simulink model "Powertrain_Mechanics_and_Dynamics"  (R2017b)
settings: Solver=VariableStepAuto  StartTime=0.0  StopTime=5  RelTol=1e-3
values from neighbouring files (symbols this model uses):
  P_2_0 = 0    [Gearbox_SLX_m.m]
  x_5_0 = 0    [Gearbox_SLX_m.m]
undefined symbols (not defined in the file or in its folder): A, b_dt, b_r, b_rg, C_d, c_roll, g, J_dt, J_r, K_dt, K_rg, M, P_3_0, P_4_0, r_g, r_r, r_w, rho, slope_out, w_6_0, x_in
settings Model: Creator=Luca  LastModifiedBy=Luca

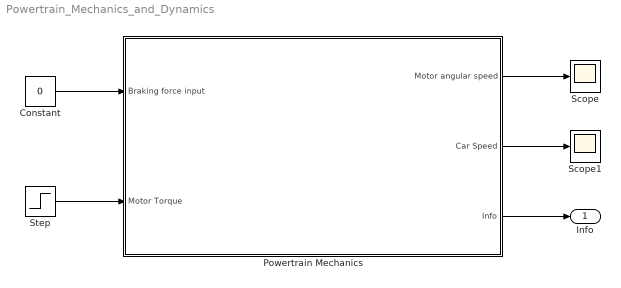
== system Powertrain_Mechanics_and_Dynamics ==
  Constant : Constant  Value=0
  Powertrain Mechanics : Subsystem
  Scope : Scope
  Scope1 : Scope
  Step : Step  After=200  SampleTime=0
  Info : Outport
  wires:
  Constant/1 -> Powertrain Mechanics/1(Braking force input)
  Step/1 -> Powertrain Mechanics/2(Motor Torque)
  Powertrain Mechanics/1(Motor angular speed) -> Scope/1
  Powertrain Mechanics/2(Car Speed) -> Scope1/1
  Powertrain Mechanics/3(Info) -> Info/1

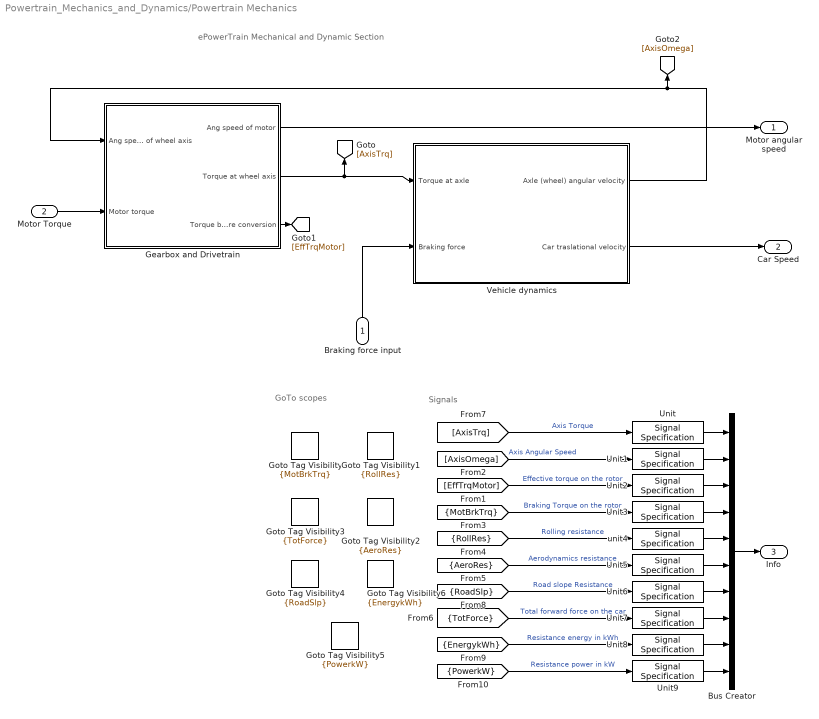
== system Powertrain_Mechanics_and_Dynamics/Powertrain Mechanics ==
  note: GoTo scopes
  note: Signals
  note: ePowerTrain Mechanical and Dynamic Section
  Braking force input : Inport
  Motor Torque : Inport  Port=2
  Bus Creator : BusCreator  Inputs=10
  Gearbox and Drivetrain : Subsystem
  Goto Tag Visibility : GotoTagVisibility  GotoTag=MotBrkTrq
  Goto Tag Visibility1 : GotoTagVisibility  GotoTag=RollRes
  Goto Tag Visibility2 : GotoTagVisibility  GotoTag=AeroRes
  Goto Tag Visibility3 : GotoTagVisibility  GotoTag=TotForce
  Goto Tag Visibility4 : GotoTagVisibility  GotoTag=RoadSlp
  Goto Tag Visibility5 : GotoTagVisibility  GotoTag=PowerkW
  Goto Tag Visibility6 : GotoTagVisibility  GotoTag=EnergykWh
  Unit : SignalSpecification  Unit=N*m
  Unit1 : SignalSpecification  Unit=rad/s
  Unit2 : SignalSpecification  Unit=N*m
  Unit3 : SignalSpecification  Unit=N*m
  Unit5 : SignalSpecification  Unit=N
  Unit6 : SignalSpecification  Unit=N
  Unit7 : SignalSpecification  Unit=N
  Unit8 : SignalSpecification  Unit=k*W*h
  Unit9 : SignalSpecification  Unit=k*W
  Vehicle dynamics : Subsystem
  unit4 : SignalSpecification  Unit=N
  Motor angular speed : Outport
  Car Speed : Outport  Port=2
  Info : Outport  Port=3
  wires:
  Vehicle dynamics/1(Axle (wheel) angular velocity) -> [AxisOmega], Gearbox and Drivetrain/1(Ang speed of wheel axis)
  Braking force input/1 -> Vehicle dynamics/2(Braking force)
  Gearbox and Drivetrain/2(Torque at wheel axis) -> Vehicle dynamics/1(Torque at axle), [AxisTrq]
  Gearbox and Drivetrain/3(Torque before conversion) -> [EffTrqMotor]
  [AxisOmega] -> Unit1/1  "Axis Angular Speed"
  [AxisTrq] -> Unit/1  "Axis Torque"
  Bus Creator/1 -> Info/1
  [RollRes] -> unit4/1  "Rolling resistance"
  Motor Torque/1 -> Gearbox and Drivetrain/2(Motor torque)
  Gearbox and Drivetrain/1(Ang speed of motor) -> Motor angular speed/1
  [AeroRes] -> Unit5/1  "Aerodynamics resistance"
  [MotBrkTrq] -> Unit3/1  "Braking Torque on the rotor"
  [TotForce] -> Unit7/1  "Total forward force on the car"
  [EffTrqMotor] -> Unit2/1  "Effective torque on the rotor"
  [RoadSlp] -> Unit6/1  "Road slope Resistance"
  Vehicle dynamics/2(Car traslational velocity) -> Car Speed/1
  [PowerkW] -> Unit9/1  "Resistance power in kW"
  [EnergykWh] -> Unit8/1  "Resistance energy in kWh"
  Unit/1 -> Bus Creator/1
  Unit1/1 -> Bus Creator/2
  Unit2/1 -> Bus Creator/3
  Unit3/1 -> Bus Creator/4
  unit4/1 -> Bus Creator/5
  Unit5/1 -> Bus Creator/6
  Unit6/1 -> Bus Creator/7
  Unit7/1 -> Bus Creator/8
  Unit8/1 -> Bus Creator/9
  Unit9/1 -> Bus Creator/10

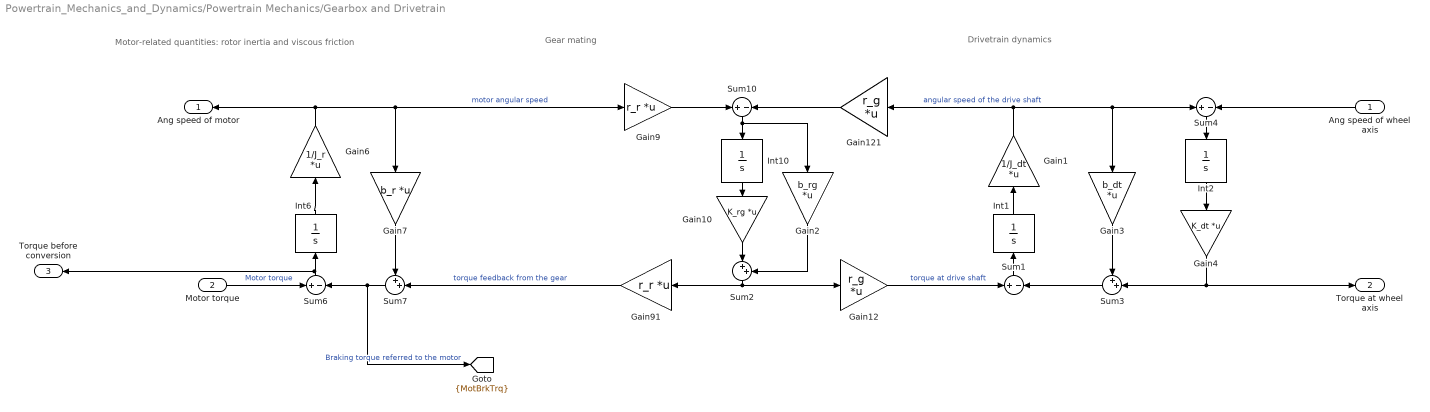
== system Powertrain_Mechanics_and_Dynamics/Powertrain Mechanics/Gearbox and Drivetrain ==
  note: Drivetrain dynamics
  note: Gear mating
  note: Motor-related quantities: rotor inertia and viscous friction
  Ang speed of wheel axis : Inport
  Motor torque : Inport  Port=2
  Gain1 : Gain  Gain=1/J_dt  Multiplication=Matrix(K*u)  SaturateOnIntegerOverflow=on  OutDataTypeStr=Inherit: Same as input  ParamDataTypeStr=Inherit: Same as input
  Gain10 : Gain  Gain=K_rg  Multiplication=Matrix(K*u)  SaturateOnIntegerOverflow=on  OutDataTypeStr=Inherit: Same as input  ParamDataTypeStr=Inherit: Same as input
  Gain12 : Gain  Gain=r_g  Multiplication=Matrix(K*u)  SaturateOnIntegerOverflow=on  OutDataTypeStr=Inherit: Same as input  ParamDataTypeStr=Inherit: Same as input
  Gain121 : Gain  Gain=r_g  Multiplication=Matrix(K*u)  SaturateOnIntegerOverflow=on  OutDataTypeStr=Inherit: Same as input  ParamDataTypeStr=Inherit: Same as input
  Gain2 : Gain  Gain=b_rg  Multiplication=Matrix(K*u)  SaturateOnIntegerOverflow=on  OutDataTypeStr=Inherit: Same as input  ParamDataTypeStr=Inherit: Same as input
  Gain3 : Gain  Gain=b_dt  Multiplication=Matrix(K*u)  SaturateOnIntegerOverflow=on  OutDataTypeStr=Inherit: Same as input  ParamDataTypeStr=Inherit: Same as input
  Gain4 : Gain  Gain=K_dt  Multiplication=Matrix(K*u)  SaturateOnIntegerOverflow=on  OutDataTypeStr=Inherit: Same as input  ParamDataTypeStr=Inherit: Same as input
  Gain6 : Gain  Gain=1/J_r  Multiplication=Matrix(K*u)  SaturateOnIntegerOverflow=on  OutDataTypeStr=Inherit: Same as input  ParamDataTypeStr=Inherit: Same as input
  Gain7 : Gain  Gain=b_r  Multiplication=Matrix(K*u)  SaturateOnIntegerOverflow=on  OutDataTypeStr=Inherit: Same as input  ParamDataTypeStr=Inherit: Same as input
  Gain9 : Gain  Gain=r_r  Multiplication=Matrix(K*u)  SaturateOnIntegerOverflow=on  OutDataTypeStr=Inherit: Same as input  ParamDataTypeStr=Inherit: Same as input
  Gain91 : Gain  Gain=r_r  Multiplication=Matrix(K*u)  SaturateOnIntegerOverflow=on  OutDataTypeStr=Inherit: Same as input  ParamDataTypeStr=Inherit: Same as input
  Int1 : Integrator  InitialCondition=P_3_0
  Int10 : Integrator  InitialCondition=x_5_0
  Int2 : Integrator  InitialCondition=w_6_0
  Int6 : Integrator  InitialCondition=P_2_0
  Sum{1,4,6,10} (4 alike) : Sum  Inputs=+|-  SaturateOnIntegerOverflow=on  InputSameDT=on  OutDataTypeStr=Inherit: Same as first input
  Sum2 : Sum  Inputs=|++  SaturateOnIntegerOverflow=on  InputSameDT=on  OutDataTypeStr=Inherit: Same as first input
  Sum3 : Sum  Inputs=++|  SaturateOnIntegerOverflow=on  InputSameDT=on  OutDataTypeStr=Inherit: Same as first input
  Sum7 : Sum  Inputs=++|  SaturateOnIntegerOverflow=on  InputSameDT=on  OutDataTypeStr=Inherit: Same as first input
  Ang speed of motor : Outport  VectorParamsAs1DForOutWhenUnconnected=on
  Torque at wheel axis : Outport  Port=2  VectorParamsAs1DForOutWhenUnconnected=on
  Torque before conversion : Outport  Port=3  VectorParamsAs1DForOutWhenUnconnected=on
  tag scope: MotBrkTrq=scoped
  wires:
  Gain91/1 -> Sum7/2  "torque feedback from the gear"
  Sum10/1 -> Gain2/1, Int10/1
  Gain6/1 -> Ang speed of motor/1, Gain9/1, Gain7/1  "motor angular speed"
  Sum7/1 -> [MotBrkTrq], Sum6/2  "Braking torque referred to the motor"
  Int6/1 -> Gain6/1
  Sum6/1 -> Torque before conversion/1, Int6/1
  Gain9/1 -> Sum10/1
  Gain7/1 -> Sum7/1
  Gain121/1 -> Sum10/2
  Sum2/1 -> Gain91/1, Gain12/1
  Gain10/1 -> Sum2/1
  Gain2/1 -> Sum2/2
  Motor torque/1 -> Sum6/1  "Motor torque"
  Int10/1 -> Gain10/1
  Gain12/1 -> Sum1/1  "torque at drive shaft"
  Sum3/1 -> Sum1/2
  Gain4/1 -> Sum3/2, Torque at wheel axis/1
  Int1/1 -> Gain1/1
  Sum1/1 -> Int1/1
  Gain1/1 -> Sum4/1, Gain3/1, Gain121/1  "angular speed of the drive shaft"
  Ang speed of wheel axis/1 -> Sum4/2
  Gain3/1 -> Sum3/1
  Int2/1 -> Gain4/1
  Sum4/1 -> Int2/1

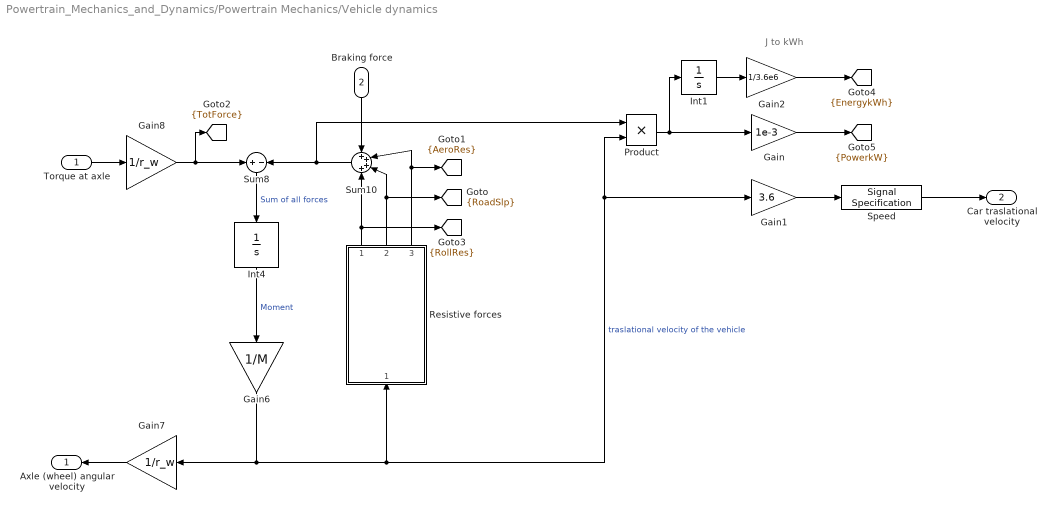
== system Powertrain_Mechanics_and_Dynamics/Powertrain Mechanics/Vehicle dynamics ==
  note: J to kWh
  Torque at axle : Inport
  Braking force : Inport  Port=2
  " Resistive forces" : Subsystem
  Gain : Gain  Gain=1e-3
  Gain1 : Gain  Gain=3.6
  Gain2 : Gain  Gain=1/3.6e6
  Gain6 : Gain  Gain=1/M  SaturateOnIntegerOverflow=on  OutDataTypeStr=Inherit: Same as input  ParamDataTypeStr=Inherit: Same as input
  Gain7 : Gain  Gain=1/r_w  SaturateOnIntegerOverflow=on  OutDataTypeStr=Inherit: Same as input  ParamDataTypeStr=Inherit: Same as input
  Gain8 : Gain  Gain=1/r_w  SaturateOnIntegerOverflow=on  OutDataTypeStr=Inherit: Same as input  ParamDataTypeStr=Inherit: Same as input
  Int1 : Integrator  InitialCondition=P_4_0
  Int4 : Integrator  InitialCondition=P_4_0
  Product : Product
  Speed : SignalSpecification  Unit=km/h
  Sum10 : Sum  Inputs=++++  SaturateOnIntegerOverflow=on  InputSameDT=on  OutDataTypeStr=Inherit: Same as first input
  Sum8 : Sum  Inputs=+|-  SaturateOnIntegerOverflow=on  InputSameDT=on  OutDataTypeStr=Inherit: Same as first input
  Axle (wheel) angular velocity : Outport
  Car traslational velocity : Outport  Port=2
  tag scope: AeroRes=scoped, EnergykWh=scoped, PowerkW=scoped, RoadSlp=scoped, RollRes=scoped, TotForce=scoped
  wires:
  Gain7/1 -> Axle (wheel) angular velocity/1
  Gain8/1 -> [TotForce], Sum8/1
  Sum8/1 -> Int4/1  "Sum of all forces"
  Gain6/1 -> Product/2, Gain1/1, " Resistive forces"/1(Traslational velocity), Gain7/1  "traslational velocity of the vehicle"
  Int4/1 -> Gain6/1  "Moment"
  Sum10/1 -> Product/1, Sum8/2
  Torque at axle/1 -> Gain8/1
  " Resistive forces"/2("  Road slope") -> Sum10/3, [RoadSlp]
  Braking force/1 -> Sum10/1
  " Resistive forces"/1(Rolling res) -> [RollRes], Sum10/4
  " Resistive forces"/3(" Drag Force") -> Sum10/2, [AeroRes]
  Product/1 -> Int1/1, Gain/1
  Int1/1 -> Gain2/1
  Gain1/1 -> Speed/1
  Speed/1 -> Car traslational velocity/1
  Gain2/1 -> [EnergykWh]
  Gain/1 -> [PowerkW]

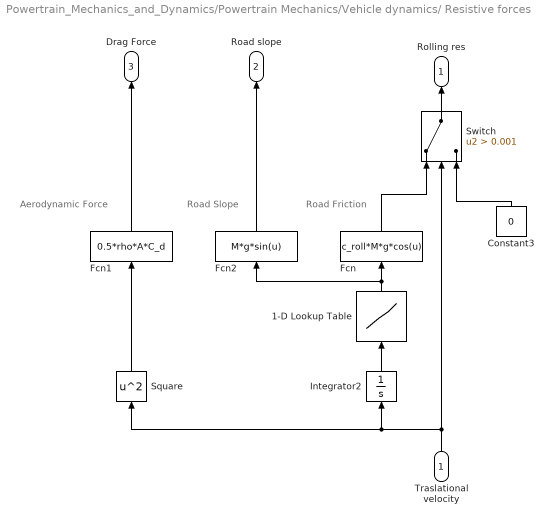
== system Powertrain_Mechanics_and_Dynamics/Powertrain Mechanics/Vehicle dynamics/ Resistive forces ==
  note: Aerodynamic Force
  note: Road Friction
  note: Road Slope
  Traslational velocity : Inport
  1-D Lookup Table : Lookup_n-D  NumberOfTableDimensions=1  BreakpointsForDimension1=x_in  Table=slope_out  InternalRulePriority=Speed  RndMeth=Simplest  InputSameDT=on
  Constant3 : Constant  Value=0
  Fcn : Fcn  Expr=c_roll*M*g*cos(u)
  Fcn1 : Fcn  Expr=0.5*rho*A*C_d
  Fcn2 : Fcn  Expr=M*g*sin(u)
  Integrator2 : Integrator
  Square : Math  Operator=square  SaturateOnIntegerOverflow=on
  Switch : Switch  Criteria=u2 > Threshold  Threshold=0.001
  Rolling res : Outport  VectorParamsAs1DForOutWhenUnconnected=on
  "  Road slope" : Outport  Port=2  VectorParamsAs1DForOutWhenUnconnected=on
  " Drag Force" : Outport  Port=3  VectorParamsAs1DForOutWhenUnconnected=on
  wires:
  Switch/1 -> Rolling res/1
  Constant3/1 -> Switch/3
  Traslational velocity/1 -> Square/1, Integrator2/1, Switch/2
  Fcn2/1 -> "  Road slope"/1
  Fcn/1 -> Switch/1
  Integrator2/1 -> 1-D Lookup Table/1
  Fcn1/1 -> " Drag Force"/1
  Square/1 -> Fcn1/1
  1-D Lookup Table/1 -> Fcn2/1, Fcn/1
